simulink model "arduino_klow"  (R2015a)
settings: Solver=ode3  StartTime=0.0  StopTime=10.0  FixedStep=1/200  RelTol=1e-3
values from neighbouring files (symbols this model uses):
  gain = -0.02    [controller_parameters.m]    (also in klowscript.m = -5)
  p1 = -200    [klowscript.m]
  p2 = 0    [klowscript.m]
  z1 = -2.5+10.47i    [klowscript.m]
  z2 = -2.5-10.47i    [klowscript.m]
libraries: PoliArd x6
settings Model: ExtModeTrigDuration=2  Creator=user  LastModifiedBy=user
settings OptimizationCC: OptimizeModelRefInitCode=on  LifeSpan=1
settings DebuggingCC: UnderspecifiedInitializationDetection=Classic  MergeDetectMultiDrivingBlocksExec=none
settings HardwareCC: ProdLargestAtomicInteger=Long  ProdLargestAtomicFloat=Double  ProdEndianess=LittleEndian  ProdHWDeviceType=ARM Compatible->ARM Cortex
settings RTWCC: SystemTargetFile=realtime.tlc  GenerateMakefile=off  TemplateMakefile=realtime.tmf  Description=Run on Target Hardware  RTWVerbose=off
settings ERTTargetCC: CombineOutputUpdateFcns=off  ExtModeTransport=3  ExtModeMexFile=ext_serial_win32_comm_rtt  ExtModeMexArgs=0 1 9600  ERTSrcFileBannerTemplate=realtime_code_template.cgt  ERTHdrFileBannerTemplate=realtime_code_template.cgt  ERTDataSrcFileTemplate=realtime_code_template.cgt  ERTDataHdrFileTemplate=realtime_code_template.cgt  ERTCustomFileTemplate=realtime_file_process.tlc

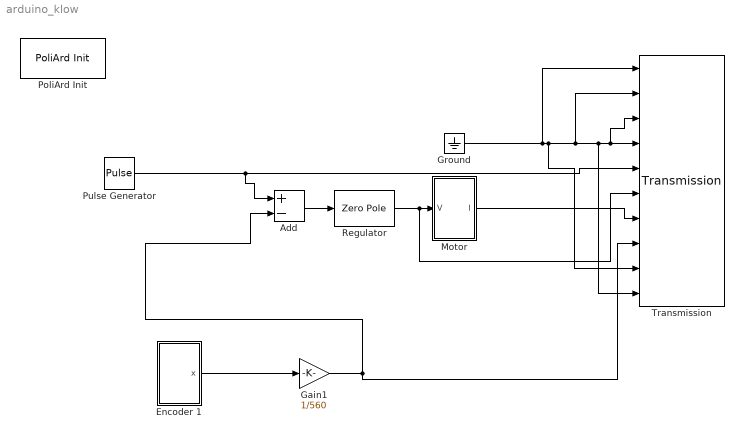
== system arduino_klow ==
  Add : Sum  Inputs=+-
  Encoder 1 : Subsystem
  Gain1 : Gain  Gain=1/560
  Ground : Ground
  Motor : Subsystem
  PoliArd Init : PoliArd/PoliArd Init
  Pulse Generator : DiscretePulseGenerator  PulseType=Time based  Period=10  PulseWidth=50  PhaseDelay=10
  Regulator : ZeroPole  Zeros=[z1,z2]  Poles=[p1,p2]  Gain=gain
  Transmission : PoliArd/Transmission  sample_freq=200  sig_to_send=6
  wires:
  Ground/1 -> Transmission/1, Transmission/9, Transmission/2, Transmission/10, Transmission/3, Transmission/4
  Motor/1(I) -> Transmission/7
  Encoder 1/1(x) -> Gain1/1
  Gain1/1 -> Add/2, Transmission/8
  Pulse Generator/1 -> Add/1, Transmission/5
  Regulator/1 -> Transmission/6, Motor/1(V)
  Add/1 -> Regulator/1

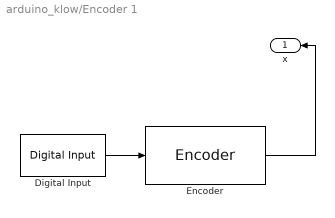
== system arduino_klow/Encoder 1 ==
  Digital Input : PoliArd/Digital Input  DI_pin=2  DIsample=1/200
  Encoder : PoliArd/Encoder  EncoderID=1  dt_enc=-1
  x : Outport
  wires:
  Digital Input/1 -> Encoder/1
  Encoder/1 -> x/1

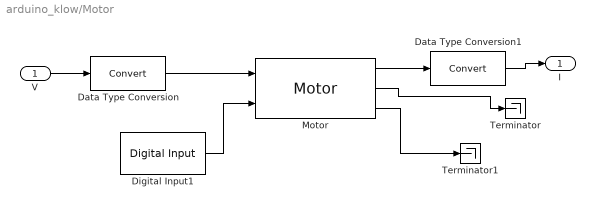
== system arduino_klow/Motor ==
  V : Inport
  Data Type Conversion : DataTypeConversion
  Data Type Conversion1 : DataTypeConversion
  Digital Input1 : PoliArd/Digital Input  DI_pin=3  DIsample=1/200
  Motor : PoliArd/Motor  MotorID=2  DC_bus_mask=12  dt_mot=1/200
  Terminator : Terminator
  Terminator1 : Terminator
  I : Outport
  wires:
  Data Type Conversion/1 -> Motor/1
  Digital Input1/1 -> Motor/2
  V/1 -> Data Type Conversion/1
  Motor/3 -> Terminator1/1
  Motor/2 -> Terminator/1
  Motor/1 -> Data Type Conversion1/1
  Data Type Conversion1/1 -> I/1
